simulink model "simpleTetheredBalloon_th"  (R2020a)
settings: Solver=VariableStepAuto  StartTime=0.0  StopTime=1000  RelTol=1e-3
libraries: simpleTetheredBalloon x1
settings Model: Creator=Ayaz  LastModifiedBy=Ayaz

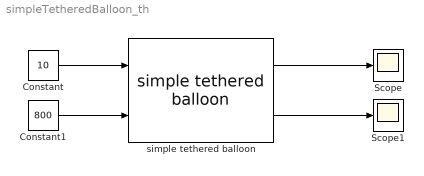
== system simpleTetheredBalloon_th ==
  Constant : Constant  Value=10
  Constant1 : Constant  Value=800
  Scope : Scope
  Scope1 : Scope
  simple tethered balloon : simpleTetheredBalloon/simple tethered balloon  rhoEnv=1.25  rhoBall=1  rBall=10  cdBall=.5  kSpring=5e6  iniAlt=600  kp=1  ki=0.1  tau=1
  wires:
  Constant/1 -> simple tethered balloon/1
  Constant1/1 -> simple tethered balloon/2
  simple tethered balloon/1 -> Scope/1
  simple tethered balloon/2 -> Scope1/1
